simulink model "linefollowing_array_solution"  (R2017a)
settings: Solver=FixedStepDiscrete  StartTime=0.0  StopTime=inf  FixedStep=0.01  RelTol=1e-3
InitFcn:
  | Ts = 0.01;
  | axleLength = 0.28;
  | wheelR = 0.052;
  | load exampleSimulationMap.mat
undefined symbols (not defined in the file): motorIp, motorSp
libraries: mobileRoboticsTrainingLib x5
settings Model: Creator=sseshadr  LastModifiedBy=shiremat

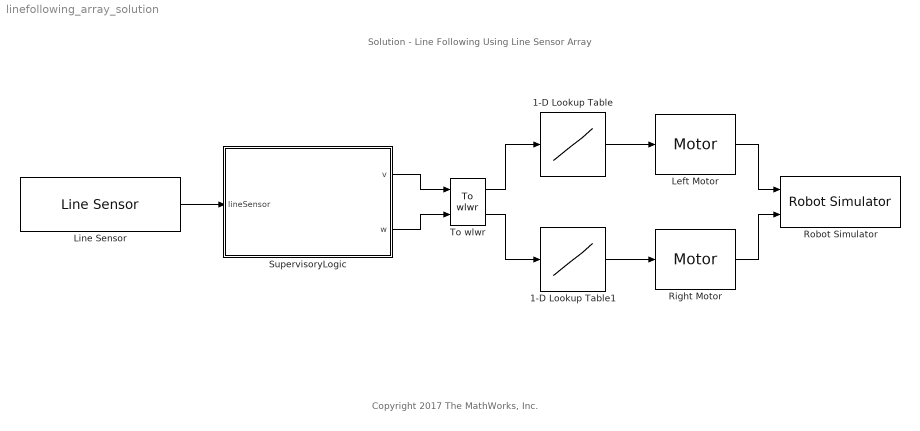
== system linefollowing_array_solution ==
  note: Solution - Line Following Using Line Sensor Array
  note: Copyright 2017 The MathWorks, Inc.
  1-D Lookup Table : Lookup_n-D  NumberOfTableDimensions=1  BreakpointsForDimension1=motorSp  Table=motorIp  ExtrapMethod=Clip  InternalRulePriority=Speed  RndMeth=Simplest  InputSameDT=on
  1-D Lookup Table1 : Lookup_n-D  NumberOfTableDimensions=1  BreakpointsForDimension1=motorSp  Table=motorIp  ExtrapMethod=Clip  InternalRulePriority=Speed  RndMeth=Simplest  InputSameDT=on
  Left Motor : mobileRoboticsTrainingLib/Motor  motorPlant=wheelMotorModel  sensorType=Speed
      settings: SourceProductName=Mobile Robotics Training Library
  Line Sensor : mobileRoboticsTrainingLib/Line Sensor  mapVariable=mapForSim  envVal=500  lineVal=0  sensOff=[0.08 0.01;0.08 0;0.08 -0.01]
      settings: SourceProductName=Mobile Robotics Training Library
  Right Motor : mobileRoboticsTrainingLib/Motor  motorPlant=wheelMotorModel  sensorType=Speed
      settings: SourceProductName=Mobile Robotics Training Library
  Robot Simulator : mobileRoboticsTrainingLib/Robot Simulator  Priority=99  mapVar=mapForSim  startX=0.6119  startY=1.3086  startTheta=0  axleLength=axleLength  wheelR=wheelR
  SupervisoryLogic : Stateflow chart  TreatAsAtomicUnit=on
  To wlwr : mobileRoboticsTrainingLib/To wlwr  axleLength=0.1  wheelR=0.05
  wires:
  Line Sensor/1 -> SupervisoryLogic/1(lineSensor)
  SupervisoryLogic/1(v) -> To wlwr/1
  SupervisoryLogic/2(w) -> To wlwr/2
  1-D Lookup Table/1 -> Left Motor/1
  1-D Lookup Table1/1 -> Right Motor/1
  Left Motor/1 -> Robot Simulator/1
  Right Motor/1 -> Robot Simulator/2
  To wlwr/1 -> 1-D Lookup Table/1
  To wlwr/2 -> 1-D Lookup Table1/1

== stateflow chart linefollowing_array_solution/SupervisoryLogic ==
  state FollowLine
    state Straight %StateB
      entry:
      v = 2.5e-2;
      w = 0;
    state BearRight %StateA
      entry:
      w = -0.2;
    state BearLeft %StateC
      entry:
      w = 0.2;
    (default) -> Straight %StateB
    Straight %StateB -> BearLeft %StateC [order 1] : [lineSensor(1) < 10]
    Straight %StateB -> BearRight %StateA [order 2] : [lineSensor(3) < 10]
    BearRight %StateA -> Straight %StateB : [lineSensor(2) < 10]
    BearLeft %StateC -> Straight %StateB : [lineSensor(2) < 10]
  (default) -> FollowLine
  data: v output; w output; lineSensor input
